simulink model "main"  (R2025b)
settings: Solver=FixedStepDiscrete  StartTime=0.0  StopTime=Inf  RelTol=1e-3  EnableMultiTasking=on
PreLoadFcn:
  | RTWConfigurationCB('preloadfcn', bdroot);
model workspace (MAT data in the model file):
  fault_count = 0
  fz_values = [0 50 100 150 200 250 300 350 400 450 500 550 ... (43 elements, 1x43)]
  k_opt_lut = [0 0 0 0 0 0 0 0 0 0 0 0 ... (4386 elements, 51x2x43)]
  mu_opt_lut = [0 0 0 0 0 0 0 0 0 0 0 0 ... (4386 elements, 51x2x43)]
undefined symbols (not defined in the file or in its folder): bit, Call, Function, ocv_lut, slope_lut, soc_lut
libraries: c2837xDlib x34, c280xlib x20, canmsglib x18, c2802xlib x12, simulink x9, slpidlib x3
(part 5 of 5)

== matlab function main/MCU Code/Subsystem/cooling_loop_fault_check2 ==
  data: i_avg_long input; cooling_loop_fault output; i_avg_short input
function cooling_loop_fault = fcn(i_avg_long, i_avg_short)
persistent fault;

if isempty(fault)
    fault = 0;
end

i_nom = 0; %Nominal current, A
i_stall = 10; %Stall current, A

if fault == 0
    if i_avg_long > (i_nom+(1-exp(-1))*(i_stall-i_nom))
        fault = 1;
    else
        fault = 0;
    end
else
    if i_avg_short < (i_nom-(1-exp(-1))*(i_nom-i_stall))
        fault = 0;
    else
        fault = 1;
    end
end

cooling_loop_fault = fault;

== matlab function main/MCU Code/MATLAB Function10 ==
  data: bpt_front_1 input; bpt_front output; bpt_front_2 input
function bpt_front = fcn(bpt_front_1,bpt_front_2)
    if abs(bpt_front_1-bpt_front_2) < 5 %some unit, size
        bpt_front = (bpt_front_1+bpt_front_2)/2;
    else
        bpt_front = max(bpt_front_1,bpt_front_2);
    end
end

== matlab function main/MCU Code/Pedals Curve/MATLAB Function ==
  data: exp input; table output
function table = fcn(exp)
table = linspace(0,1,100).^exp;

== matlab function main/MCU Code/TC Controller/MATLAB Function ==
  data: a_y input; F_Y output
function F_Y = fcn(a_y)
m = 250+68; %Mass with driver weight
a = 1.530/2; %Distance cg to front axle with load distribution of 0.5
h = 0.249; %Height of CG
l = 1.530; %Length of wheelbase

F_Y = (a/l)*m*a_y;

== matlab function main/MCU Code/TC Controller/MATLAB Function10 ==
  data: a_x input; F_Z output; a_y input
function F_Z = fcn(a_x, a_y)
m = 250+68; %Mass with driver weight
a = 1.530/2; %Distance cg to front axle with load distribution of 0.5
h = 0.249; %Height of CG
l = 1.530; %Length of wheelbase
tw = 1.2; %Track width
roll_stiffness_r = 0.3482;
F_Z = (1/2)*m*(a+h*a_x)/(l);
%F_Z_out = 1/2*((m*a)/l + (m*h*a_x)/l) + (m*abs(a_y)*h)/tw;
%F_Z_in = 1/2*((m*a)/l + (m*h*a_x)/l) - (m*abs(a_y)*h)/tw;
%F_Z = min(F_Z_out,F_Z_in);

== matlab function main/MCU Code/TC Controller/Subsystem/MATLAB Function1 ==
  data: fz input; fy input; k_table input; k_opt output
function k_opt = fcn(fz,fy,k_table)
    if fz == 0
        k_opt = 0;
    else
        k_opt = interp1(double(k_table(:,1))/10000,double(k_table(:,2))/100,fy,'linear','extrap');
    end

== stateflow chart main/MCU Code/Chart1 ==
  state REGEN_AVAILABLE
    Regen_State = 2;
  state REGEN_OFF
    Regen_State = 0;
  state REGEN_NOT_AVAILABLE
    Regen_State = 1;
  (default) -> REGEN_OFF
  REGEN_AVAILABLE -> REGEN_OFF [order 1] : [~regen_switch]
  REGEN_NOT_AVAILABLE -> REGEN_OFF [order 1] : [~regen_switch]
  REGEN_OFF -> REGEN_NOT_AVAILABLE : [regen_switch]
  REGEN_NOT_AVAILABLE -> REGEN_AVAILABLE [order 2] : [v_fr > 700 && bpt_f > 28 && bpt_r > 28 && voltage < 255 && pedals <= 0.0 && brake_bias_good]
  REGEN_AVAILABLE -> REGEN_NOT_AVAILABLE [order 2] : [v_fr <= 700 || bpt_f <= 28 || bpt_r <= 28 || voltage >= 255 || pedals > 0.0 || ~brake_bias_good]
  data: v_fr input; bpt_f input; bpt_r input; pedals input; voltage input; regen_switch input; Regen_State output double; brake_bias_good input

== matlab function main/MCU Code/Subsystem1/MATLAB Function5 ==
  data: z input; i_dis output; sig_z input; i_chg output; ocv_lut parameter; slope_lut parameter; soc_lut parameter
function [i_dis,i_chg] = i_calc(z,sig_z,ocv_lut, slope_lut, soc_lut)
    z_min = 0.2; %SOC min
    z_max = 0.9; %SOC max
    v_min = 2.4; %1 Cell Voltage Min [V]
    v_max = 4.167; %1 Cell Voltage Max [V]
    dt = 1; %Time Step
    C = 10.4; %Capacity in [Amp-Hours]
    r_dis = 0.0035; %Dicharge Internal Resistance [Ohms]
    r_chg = 0.0035;  %Charge Internal Resistance [Ohms]
    nu = 1; %Efficiency
    i_max = 140; %Max Current [Amps]
    i_min = -140; %Min Current [Amps]
    

    i_dis_soc = ((z-3*sig_z) - z_min)/(dt/C);
    i_chg_soc = ((z-3*sig_z) - z_max)/(dt*nu/C);
    
    ocv = interp1(soc_lut,ocv_lut, z, 'linear');
    ke = interp1(soc_lut, slope_lut, z, 'linear');

    low = z < 0.05;
    high = z > 0.95;
    
    ocv(low) = 2.5;
    ocv(high) = 4.2;

    ke(low) = 137.4725;
    ke(high) = 4;
  
    i_dis_volt = (ocv - v_min)./((dt/C)*ke+r_dis);
    i_chg_volt = (ocv - v_max)./((dt/C)*ke+r_chg);
 
    i_dis = min(i_max,min(min(i_dis_soc),min(i_dis_volt)));
    i_chg = max(i_min,max(max(i_chg_soc),max(i_chg_volt)));
end

== matlab function main/MCU Code/Subsystem1/MATLAB Function14 ==
  data: i_dis input; p_dis_max output; i_chg input; z input; p_chg_min output; soc_lut parameter; ocv_lut parameter
function [p_dis_max,p_chg_min] = power_calc(i_dis,i_chg,z,soc_lut, ocv_lut)
    dt = 1; %Time Step
    C = 10.4; %Capacity [Amp-Hours]
    np = 4; %Number of parallel cells
    r_dis = 0.0035; %Discharge Internal Resistance [Ohms]
    r_chg = 0.0035; %Charge Internal Resistance [Ohms]

    ocv_dis = interp1(soc_lut,ocv_lut, (z-i_dis*(dt/C)), 'linear');
    ocv_chg = interp1(soc_lut,ocv_lut, (z-i_chg*(dt/C)), 'linear');

    low = z < 0.05;
    high = z > 0.95;
    
    ocv_dis(low) = 2.5;
    ocv_dis(high) = 4.2;

    ocv_chg(low) = 2.5;
    ocv_chg(high) = 4.2;
   
    p_dis_max = np*sum(i_dis*(ocv_dis-r_dis*i_dis)); %Sums all cells
    p_chg_min = np*sum(i_chg*(ocv_chg-r_chg*i_chg));
end

== matlab function main/MCU Code/MATLAB Function14 ==
  data: bsm_discharge input; discharge output; length input
function discharge  = fcn(bsm_discharge, length)

% if timeout
%     out = -1; % timeout in TS state CAN signal
persistent timeout;
if isempty(timeout)
    timeout = 0;
end

if length == 0
    timeout = timeout + 1;
else
    timeout = 0;
end

if timeout > 200
    discharge = 0;
else
    discharge = bsm_discharge;
end

== matlab function main/MCU Code/TC Controller/Subsystem/MATLAB Function4 ==
  data: FZ input; FZ_value output; j output; fz_values parameter
function [FZ_value,j] = fcn(FZ,fz_values)
  FZ = FZ*1000;
  m = 10000;
  index = 1;
  for i = 1:numel(fz_values)
      delta = abs(FZ - fz_values(i));
      if delta < m
          m = delta;
          index = i;
      else
          m = m;
      end
  end
    FZ_value = fz_values(index);
    j = index;
end

== matlab function main/MCU Code/TC Controller/Subsystem/MATLAB Function2 ==
  data: mu_table input; fz input; mu_x output; fy input
function mu_x = fcn(mu_table,fz, fy)
    if fz == 0
        mu_x = 0;
    else
        mu_x = interp1(double(mu_table(:,1))/10000,double(mu_table(:,2))/1000,fy,"linear","extrap");
    end

== matlab function main/Subsystem/MATLAB Function1 ==
  data: u input; y output
function y = fcn(u)
if u==1
    y = 1;
else
    y = 0;
end

== matlab function main/MCU Code/MATLAB Function12 ==
  data: TC_switch input; driver_input_ctrl output; Driver_Torque_switch input; mcu_input_ctrl output; Regen_switch input
function [driver_input_ctrl,mcu_input_ctrl] = fcn(TC_switch,Driver_Torque_switch,Regen_switch)
    if TC_switch == 1 && Regen_switch == 0
        mcu_input_ctrl = 1;
    elseif TC_switch == 0 && Regen_switch == 1
        mcu_input_ctrl = 2;
    elseif TC_switch == 1 && Regen_switch == 1
        mcu_input_ctrl = 3;
    else
        mcu_input_ctrl = 0;
    end
    
    if Driver_Torque_switch == 0
        driver_input_ctrl = 1;
    else
        driver_input_ctrl = 0;
    end

== matlab function main/MCU Code/MATLAB Function2 ==
  data: bpt_f_1 input; bpt_f_1_bar output; bpt_f_2 input; bpt_f_2_bar output
function [bpt_f_1_bar,bpt_f_2_bar] = fcn(bpt_f_1,bpt_f_2)
bpt_f_1_bar = double((((single(bpt_f_1)/4095)*3.3*4)-0.5)*25);
bpt_f_2_bar = double((((single(bpt_f_2)/4095)*3.3*4)-0.5)*25);

== matlab function main/MCU Code/Regen_Direct_Calculation/MATLAB Function ==
  data: F_bf output; Pr_f input; F_br output; Pr_r input
function [F_bf,F_br] = fcn(Pr_f,Pr_r)
mu = 0.410;
r_rotor = 76.96e-3; %m, effective rotor radius
r_tire = 203.2e-3; %m
A_r = 1816e-6; %m^2
%psi_to_bar = 1/14.503;
%maybe ((1/BB_e)-1), MIT paper, now is just some variable 0 to 1 minus 1
F_br = (2*mu*(r_rotor/r_tire)*A_r*Pr_r)*(100000);
F_bf = (2*mu*(r_rotor/r_tire)*A_r*Pr_f)*(100000);

== matlab function main/MCU Code/Regen_Direct_Calculation/MATLAB Function1 ==
  data: F_rg output; F_bf input; F_br input; breaking_bias input; b output
function [F_rg, b]= fcn(F_bf,F_br,breaking_bias)

F_rg = F_bf/breaking_bias - (F_bf + F_br);
b=F_bf/(F_rg+F_bf+F_br);

== matlab function main/MCU Code/Regen_Direct_Calculation/MATLAB Function2 ==
  data: F_bf output; Pr_f input; F_br output; Pr_r input
function [F_bf,F_br] = fcn(Pr_f,Pr_r)
mu = 0.410;
r_rotor = 76.96e-3; %m, effective rotor radius
r_tire = 203.2e-3; %m
A_r = 1816e-6; %m^2
%psi_to_bar = 1/14.503;
%maybe ((1/BB_e)-1), MIT paper, now is just some variable 0 to 1 minus 1
F_br = (2*mu*(r_rotor/r_tire)*A_r*Pr_r)*(100000);
F_bf = (2*mu*(r_rotor/r_tire)*A_r*Pr_f)*(100000);

== matlab function main/MCU Code/Power Limiting1/MATLAB Function ==
  data: Id input; P_r output; Iq input
function P_r = fcn(Id,Iq)

P_r = 3/2*0.006*(Id^2+Iq^2);

== matlab function main/MCU Code/Regen_Direct_Calculation/MATLAB Function4 ==
  data: F_br input; breaking_bias output; F_bf input; F_rg input
function breaking_bias = fcn( F_br,F_bf,F_rg)

breaking_bias = F_bf/(F_br+F_bf+F_rg);

== matlab function main/Subsystem/MATLAB Function ==
  data: t input; t_hit input; rtm output; sdc_low input; sdc_high input
function rtm = fcn(t, t_hit, sdc_low, sdc_high)

persistent time_latch;
persistent check_immediate;
persistent check_wait;
persistent out;
persistent counter;

if isempty(time_latch)
    time_latch = 0;
end

if isempty(check_immediate)
    check_immediate = false;
end

if isempty(check_wait)
    check_wait = false;
end

if isempty(out)
    out = false;
end

if isempty(counter)
    counter = false
end

if sdc_high
    check_immediate = true;
    if counter == false
        counter = true
    end
end

if sdc_low & counter
    time_latch = t;
    check_wait = true;
end
%Wait 0.0045 seconds to change rtm signal
if (check_immediate)
    out = true;
    check_immediate = false;
end

%Wait 0.0045 seconds to change rtm signal
if (check_wait & t-time_latch >= 8)
    out = false;
    check_wait = false;
end

rtm = out;

== matlab function main/In Signals/MATLAB Function ==
  data: hit input; bspd_in input; bspd output; t input
function bspd = fcn(hit, bspd_in, t)
persistent time_fault;
persistent check;

if isempty(time_fault)
    time_fault = 0;
end

if isempty(check)
    check = false;
end

%Check for BSPD latch
if (hit)
    time_fault = t;
    check = true;
end

%Force BSPD to stay 0 for 0.02 seconds
if check & (t-time_fault < 0.02)
    bspd = 0;
else %Listen to BSPD actual
    bspd = bspd_in;
    check = false;
end
